simulink model "DvrSimKeybdCircuit_cs_old"  (R2016a)
settings: Solver=ode5  SolverMode=SingleTasking  StartTime=0.0  StopTime=inf  FixedStep=1/1000  RelTol=1e-3
PreLoadFcn:
  | mbxruntime.callbacks.PreLoadFcn(bdroot);
PostLoadFcn:
  | mbxruntime.callbacks.PostLoadFcn(bdroot);
InitFcn:
  | mbxruntime.callbacks.InitFcn(bdroot);
StartFcn:
  | mbxruntime.callbacks.StartFcn(bdroot);
StopFcn:
  | mbxruntime.callbacks.StopFcn(bdroot);
model workspace (MAT data in the model file):
  mbox_table : struct (value not decoded)
  model_closed = 0
  sim_status = 0
undefined symbols (not defined in the file or in its folder): BMotor1, BMotor2, BrkDelayTime, DControlB, Delay1, Delay2, DiscIntNeverNeededParam, IControlB, JMotor1, JMotor2, PControlB, PreScanCarSimLoadFcn, ratioGearF, ratioGearR, TorqDelayTime, Tstep
undefined symbols (not defined in the file): SteeringColumn, SteeringWheel, WheelL0, WheelL1, WheelR0, WheelR1
libraries: simulink x12, simulink_extras x5, MyLib x3, PreScanSimulinkLibrary x3, Solver_SF x2, pil_lib x1, PreScanUsefulBlocks x1
(part 2 of 9)

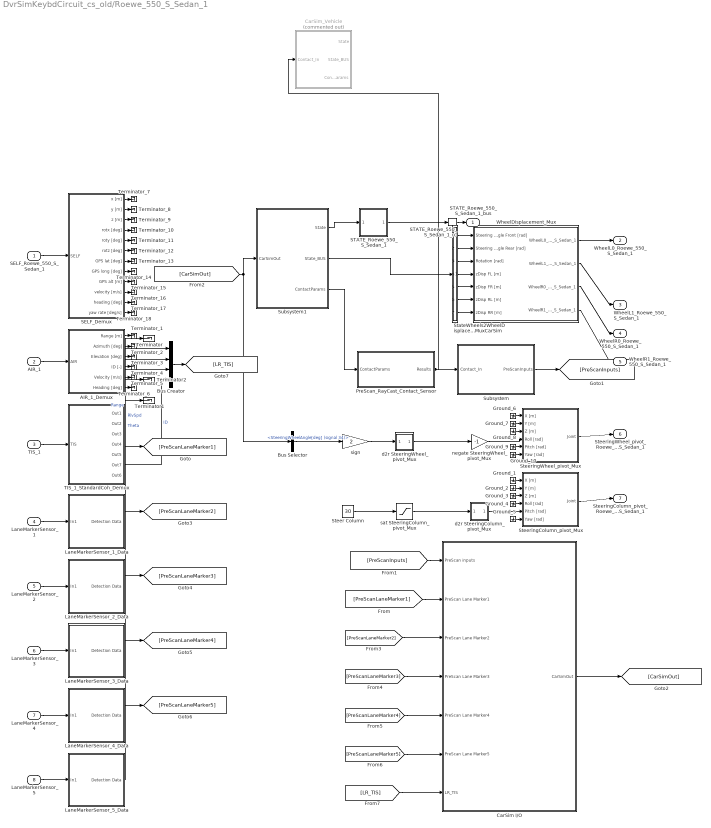
== system DvrSimKeybdCircuit_cs_old/Roewe_550_S_Sedan_1 ==
  SELF_Roewe_550_S_Sedan_1 : Inport  Tag=inport/SelfPort  OutDataTypeStr=Bus: PRESCAN_SELFSENSORDATA  PortDimensions=1  SampleTime=50/1000  BusOutputAsStruct=on
  AIR_1 : Inport  Tag=inport/AIR  Port=2  OutDataTypeStr=Bus: PRESCAN_AIRSENSORMESSAGE  PortDimensions=1  SampleTime=50/1000  BusOutputAsStruct=on
  TIS_1 : Inport  Tag=inport/TIS  Port=3  OutDataTypeStr=Bus: PRESCAN_SCANNERSENSOR_MESSAGE  PortDimensions=1  SampleTime=1/20  BusOutputAsStruct=on
  LaneMarkerSensor_1 : Inport  Tag=inport/LaneMarker  Port=4  OutDataTypeStr=Bus: PRESCAN_LANEMARKER_MESSAGE  PortDimensions=4  SampleTime=1/20  BusOutputAsStruct=on
  LaneMarkerSensor_2 : Inport  Tag=inport/LaneMarker  Port=5  OutDataTypeStr=Bus: PRESCAN_LANEMARKER_MESSAGE  PortDimensions=4  SampleTime=1/20  BusOutputAsStruct=on
  LaneMarkerSensor_3 : Inport  Tag=inport/LaneMarker  Port=6  OutDataTypeStr=Bus: PRESCAN_LANEMARKER_MESSAGE  PortDimensions=4  SampleTime=1/20  BusOutputAsStruct=on
  LaneMarkerSensor_4 : Inport  Tag=inport/LaneMarker  Port=7  OutDataTypeStr=Bus: PRESCAN_LANEMARKER_MESSAGE  PortDimensions=4  SampleTime=1/20  BusOutputAsStruct=on
  LaneMarkerSensor_5 : Inport  Tag=inport/LaneMarker  Port=8  OutDataTypeStr=Bus: PRESCAN_LANEMARKER_MESSAGE  PortDimensions=4  SampleTime=1/20  BusOutputAsStruct=on
  AIR_1_Demux : Subsystem  Tag=demux/AIR  mask(PreScan Demux Block: AIR){DetectionType=Center, detectableObjects=1}
      mask prompts: DetectionType "Detection Type"; detectableObjects "Max. detectable objects"
      mask help:
      | The Actor Information Receiver sensor provides a fast, simple and generic detection solution which is not tied up to a specific technology and can be used for scenarios in which a simple sensor is needed.
      |
      | For more information, please click Help.
      mask init:
      | switch DetectionType
      |     case 1
      |         DetectionTypeStr = 'Center';
      |     case 2
      |         DetectionTypeStr = 'BBox';
      |     case 3
      |         DetectionTypeStr = 'CoG';
      |     otherwise
      |         DetectionTypeStr = 'Unknown';
      | end
      settings: DeleteFcn=PreScanBlockDeleteFcn;
      mask Help: eval('openHelp(413)')
      mask TypeOptions DetectionType: Center | BBox | CoG
      mask Display:
      | disp(char('Det. type:         ',['{\it',DetectionTypeStr,'}']),'texmode','on')
      | port_label('output',1,'Range [m]')
      | port_label('output',2,'{\theta} [deg]','texmode','on')
      | port_label('output',3,'{\phi} [deg]','texmode','on')
      | port_label('output',4,'ID [-]','texmode','on')
      | port_label('output',5,'Velocity [m/s]','texmode','on')
      | port_label('output',6,'Heading [deg]','texmode','on')
  Bus Creator : BusCreator  Inputs=4
  Bus Selector : BusSelector  OutputSignals=SteeringWheelAngle[deg] (signal 34)
  CarSim I/O : Subsystem
  CarSim_Vehicle : Subsystem  Tag=UserSpecified_Subsys  Description=..\..\..\Program Files (x86)\CarSim201601_Data\Extensions\Simulink\CarSim_VehicleDynamics.mdl  Commented=on  LoadFcn=PreScanCarSimLoadFcn();  mask(User specified subsystem){update=off, sourcefilename=..\..\..\Program Files (x86)\CarSim201601_Data\Extensions\Simulink\CarSim_VehicleDynamics.mdl}
      mask prompts: update "Update (default: not checked)"; sourcefilename "Source file name"
      mask help:
      | A User-specified model may be selected as Controller or Dynamics of the vehicle. PreScan will copy the contents of the User-specified model into the user-specified model block.
      |
      | If update checkbox is checked the current user-specified model block will be deleted and will be REPLACED by (new) user specified model blocks. So, the current user specified model elements will be lost.
      |
      | Warning: If a new user-specified model is selected in the GUI, the user-specified model will be replaced.
      settings: DeleteFcn=PreScanBlockDeleteFcn;
      mask Help: eval('openHelp(227)')
      mask Display: userSpecifiedDynamics_mask_display();
  Ground_{1..10} (10 alike) : Ground
  LaneMarkerSensor_1_Data : Subsystem  Tag=demux/LaneMarkerSensor  mask{NUMBEROFSLICES=4, TimeStep=1/20}
      mask prompts: NUMBEROFSLICES "Number of slices"; TimeStep "Auto Assigned: Time Step [s]"
      mask Help: eval('openHelp(2301)')
  LaneMarkerSensor_2_Data : Subsystem  Tag=demux/LaneMarkerSensor  mask{NUMBEROFSLICES=4, TimeStep=1/20}
      mask prompts: NUMBEROFSLICES "Number of slices"; TimeStep "Auto Assigned: Time Step [s]"
      mask Help: eval('openHelp(2301)')
  LaneMarkerSensor_3_Data : Subsystem  Tag=demux/LaneMarkerSensor  mask{NUMBEROFSLICES=4, TimeStep=1/20}
      mask prompts: NUMBEROFSLICES "Number of slices"; TimeStep "Auto Assigned: Time Step [s]"
      mask Help: eval('openHelp(2301)')
  LaneMarkerSensor_4_Data : Subsystem  Tag=demux/LaneMarkerSensor  mask{NUMBEROFSLICES=4, TimeStep=1/20}
      mask prompts: NUMBEROFSLICES "Number of slices"; TimeStep "Auto Assigned: Time Step [s]"
      mask Help: eval('openHelp(2301)')
  LaneMarkerSensor_5_Data : Subsystem  Tag=demux/LaneMarkerSensor  mask{NUMBEROFSLICES=4, TimeStep=1/20}
      mask prompts: NUMBEROFSLICES "Number of slices"; TimeStep "Auto Assigned: Time Step [s]"
      mask Help: eval('openHelp(2301)')
  PreScan_RayCast_Contact_Sensor : Subsystem  Tag=PreScan_RayCast_Contact_Sensor  LoadFcn=|  mask(PreScan Block: PreScan RayCast Contact Sensor){x0=1005.0825, y0=379.7545, z0=1.22, Roll0=0, Pitch0=0, Yaw0=180, wheelRadius=0.44999998807907104, hcog=0.53, b=2.7000000476837158, TimeStep=-1}
      | load PrescanXYZData;
      | load PrescanRPYData;
      | load PrescanQuatData;
      | load PrescanAxisAngleData;
      | load PrescanPoseData;
      | load PrescanPoseQData;
      | load PrescanPoseAData;
      | load PrescanWheelContactData;
      mask prompts: x0 "Ini x-position VEHICLE wrt GLOBAL axis system [m]"; y0 "Ini y-position VEHICLE wrt GLOBAL axis system [m]"; z0 "Ini z-position VEHICLE wrt GLOBAL axis system [m]"; Roll0 "Ini roll-angle BODY wrt VEHICLE axis system [deg]"; Pitch0 "Ini pitch-angle BODY wrt VEHICLE axis system [deg]"; Yaw0 "Ini yaw-angle VEHICLE wrt GLOBAL axis system [deg]"; wheelRadius "Wheel Radius [m]"; hcog "Dynamics: hCoG [m]"; b "Dynamics: b [m]"; TimeStep "Time Step [s]"
      mask help:
      | This block encapsulates the base Contact sensor.
      |
      | It takes input parameters from the PreScan 3D vehicle dynamics block and outputs contact results.
      mask Help: eval('openHelp(251)')
  SELF_Demux : Subsystem  Tag=demux/SelfPort  mask(PreScan Demux Block:){}
      mask help:
      | The SELF port shows (state) information of the actor itself. The outputs are position in the experiment's axis system and the GPS coordinates, and the object's absolute velocity and compass heading.
      |
      | For more information, please click Help.
      settings: DeleteFcn=PreScanBlockDeleteFcn;
      mask Help: eval('openHelp(462)')
      mask Display:
      | port_label('output',1,'x [m]')
      | port_label('output',2,'y [m]')
      | port_label('output',3,'z [m]','texmode','on')
      | port_label('output',4,'Rotx [deg]','texmode','on')
      | port_label('output',5,'Roty [deg]','texmode','on')
      | port_label('output',6,'Rotz [deg]','texmode','on')
      | port_label('output',7,'GPS lat [deg]','texmode','on')
      | port_label('output',8,'GPS long [deg]','texmode','on')
      | port_label('output',9,'GPS alt [m]','texmode','on')
      | port_label('output',10,'Velocity [m/s]')
      | port_label('output',11,'Heading [deg]')
      | port_label('output',12,'Yaw rate [deg/s]')
  STATE_Roewe_550_S_Sedan_1 : Subsystem  Tag=mux/StatePort  Priority=0  LoadFcn=load PrescanStateActuatorData  mask(PreScan Sink Block: State){x0=1005.0825, y0=379.7545, z0=1.22, Roll0=0, Pitch0=0, Yaw0=180, TimeStep=1/1000}
      mask prompts: x0 "Ini x-position VEHICLE wrt GLOBAL axis system [m]"; y0 "Ini y-position VEHICLE wrt GLOBAL axis system [m]"; z0 "Ini z-position VEHICLE wrt GLOBAL axis system [m]"; Roll0 "Ini roll-angle BODY wrt VEHICLE axis system [deg]"; Pitch0 "Ini pitch-angle BODY wrt VEHICLE axis system [deg]"; Yaw0 "Ini yaw-angle VEHICLE wrt GLOBAL axis system [deg]"; TimeStep "Auto-Assigned: Upload Period [s]"
      mask help:
      | The Actor State contains a vector signal of size (9x1), containing the following signals:
      |
      | -  Position                  (x,y,z)                                     [m]
      | -  Velocity                  (vx,vy,vz)                               [m/s]
      | -  Angles                    (Roll, Pitch, Yaw)                   [rad]
      |
      | The Actor state is defined in the global axis system.
      | The state is superponed on the Initial position defined in the GUI.
      |
      | For more information, please click Help.
      settings: DeleteFcn=PreScanBlockDeleteFcn;
      mask Help: eval('openHelp(222)')
      mask Display: image(imread('State.png'))
  STATE_Roewe_550_S_Sedan_1_rc : RateTransition  Tag=mux_rc/StatePort  OutPortSampleTimeOpt=Inherit
  StateWheels2WheelDisplacementMuxCarSim : Subsystem  Tag=StateWheels2WheelDisplacementMuxCarSim  mask(PreScan Utility Block:){}
      mask help: This block selects the CarSim wheels displacement and rotation.
      settings: DeleteFcn=PreScanBlockDeleteFcn;
  Steer Column : Constant  Value=30
  SteeringColumn_pivot_Mux : Subsystem  Tag=mux/Joint  mask(PreScan Mux Block){DisplayName=SteeringColumn}
      mask prompts: DisplayName "Display Name"
      mask help:
      | This block simulates a generic joint used for generic models. This joint can be enabled/disabled from the GUI.
      |
      | For more information, please click Help.
      settings: DeleteFcn=PreScanBlockDeleteFcn;
      mask Help: eval('openHelp(254)')
  SteeringWheel_pivot_Mux : Subsystem  Tag=mux/Joint  mask(PreScan Mux Block){DisplayName=SteeringWheel}
      mask prompts: DisplayName "Display Name"
      mask help:
      | This block simulates a generic joint used for generic models. This joint can be enabled/disabled from the GUI.
      |
      | For more information, please click Help.
      settings: DeleteFcn=PreScanBlockDeleteFcn;
      mask Help: eval('openHelp(254)')
  Subsystem : Subsystem
  Subsystem1 : Subsystem
  TIS_1_StandardCoh_Demux : Subsystem  Tag=demux/TIS/StandardCoh  TreatAsAtomicUnit=on  mask(PreScan Demux Block: TIS){MAXMESSAGES=1}
      mask prompts: MAXMESSAGES "Number of Objects"
      mask Help: eval('openHelp(449)')
      mask Display:
      | port_label('input',1,'TIS')
      | port_label('output',1,'Beam ID [-]')
      | port_label('output',2,'Range [m]')
      | port_label('output',3,'DopplerVelocity [m/s]')
      | port_label('output',4,'{\theta} [deg]','texmode','on')
      | port_label('output',5,'{\phi} [deg]','texmode','on')
      | port_label('output',6,'Target ID [-]','texmode','on')
      | port_label('output',7,'TIS Data','texmode','on')
  Terminator : Terminator
  Terminator1 : Terminator
  Terminator2 : Terminator
  Terminator_{1..18} (18 alike) : Terminator
  WheelDisplacement_Mux : Subsystem  Tag=mux/JointGroup  mask(JointGroup){}
      mask help:
      | The JointGroup allows to control several Joints in one go, as defined for this particular model.
      | For more information, look in the PreScan manual in the section "Model Preparation Tool" -> "Joint Groups"
      |
      | For more information on the Joints simulink interface, press Help.
      mask Help: eval('openHelp(254)')
  d2r SteeringColumn_pivot_Mux : Subsystem  mask(DegreesToRadians){}
      mask help: SimulinkBlocks:simulink_extras:DegreesToRadians_MD
      mask Help: web([docroot '/simulink/ref_extras/degreestoradians.html'])
      mask Display: disp('D2R')
  d2r SteeringWheel_pivot_Mux : Subsystem  mask(DegreesToRadians){}
      mask help: SimulinkBlocks:simulink_extras:DegreesToRadians_MD
      mask Help: web([docroot '/simulink/ref_extras/degreestoradians.html'])
      mask Display: disp('D2R')
  negate SteeringWheel_pivot_Mux : Gain  Gain=-1
  sat SteeringColumn_pivot_Mux : Saturate  UpperLimit=30  LowerLimit=-5
  sign : Gain  Gain=2
  STATE_Roewe_550_S_Sedan_1_bus : Outport  Tag=outport/StatePort  OutDataTypeStr=Bus: PRESCAN_STATEACTUATORDATA  PortDimensions=1  SampleTime=50/1000
  WheelL0_Roewe_550_S_Sedan_1 : Outport  Tag=outport/JointActuator  Port=2  OutDataTypeStr=Bus: PRESCAN_POSE_DATA  SampleTime=50/1000
  WheelL1_Roewe_550_S_Sedan_1 : Outport  Tag=outport/JointActuator  Port=3  OutDataTypeStr=Bus: PRESCAN_POSE_DATA  SampleTime=50/1000
  WheelR0_Roewe_550_S_Sedan_1 : Outport  Tag=outport/JointActuator  Port=4  OutDataTypeStr=Bus: PRESCAN_POSE_DATA  SampleTime=50/1000
  WheelR1_Roewe_550_S_Sedan_1 : Outport  Tag=outport/JointActuator  Port=5  OutDataTypeStr=Bus: PRESCAN_POSE_DATA  SampleTime=50/1000
  SteeringWheel_pivot_Roewe_550_S_Sedan_1 : Outport  Tag=outport/JointActuator  Port=6  OutDataTypeStr=Bus: PRESCAN_POSE_DATA  SampleTime=50/1000
  SteeringColumn_pivot_Roewe_550_S_Sedan_1 : Outport  Tag=outport/JointActuator  Port=7  OutDataTypeStr=Bus: PRESCAN_POSE_DATA  SampleTime=50/1000
  wires:
  LaneMarkerSensor_1_Data/1(Detection Data) -> [PreScanLaneMarker1]
  LaneMarkerSensor_2_Data/1(Detection Data) -> [PreScanLaneMarker2]
  LaneMarkerSensor_3_Data/1(Detection Data) -> [PreScanLaneMarker3]
  LaneMarkerSensor_4_Data/1(Detection Data) -> [PreScanLaneMarker4]
  [PreScanLaneMarker1] -> CarSim I/O/2(PreScan Lane Marker1)
  [PreScanInputs] -> CarSim I/O/1(PreScan inputs)
  Subsystem/1(PreScanInputs) -> [PreScanInputs]
  [CarSimOut] -> Bus Selector/1, Subsystem1/1(CarSimOut)
  PreScan_RayCast_Contact_Sensor/1(Results) -> Subsystem/1(Contact_In), CarSim_Vehicle/1(Contact_In)
  Subsystem1/3(ContactParams) -> PreScan_RayCast_Contact_Sensor/1(ContactParams)
  Subsystem1/1(State) -> STATE_Roewe_550_S_Sedan_1/1(State)
  Subsystem1/2(State_BUS) -> StateWheels2WheelDisplacementMuxCarSim/1(StateWheels)
  CarSim I/O/1(CarSimOut) -> [CarSimOut]
  [PreScanLaneMarker2] -> CarSim I/O/3(PreScan Lane Marker2)
  [PreScanLaneMarker3] -> CarSim I/O/4(PreScan Lane Marker3)
  [PreScanLaneMarker4] -> CarSim I/O/5(PreScan Lane Marker4)
  [PreScanLaneMarker5] -> CarSim I/O/6(PreScan Lane Marker5)
  negate SteeringWheel_pivot_Mux/1 -> SteeringWheel_pivot_Mux/4(Roll [rad])
  d2r SteeringWheel_pivot_Mux/1(Radians out) -> negate SteeringWheel_pivot_Mux/1
  Bus Selector/1 -> sign/1  "<SteeringWheelAngle[deg] (signal 34)>"
  sign/1 -> d2r SteeringWheel_pivot_Mux/1(Degrees in)
  d2r SteeringColumn_pivot_Mux/1(Radians out) -> SteeringColumn_pivot_Mux/5(Pitch [rad])
  sat SteeringColumn_pivot_Mux/1 -> d2r SteeringColumn_pivot_Mux/1(Degrees in)
  Steer Column/1 -> sat SteeringColumn_pivot_Mux/1
  LaneMarkerSensor_5_Data/1(Detection Data) -> [PreScanLaneMarker5]
  TIS_1_StandardCoh_Demux/1(Out1) -> Terminator/1
  TIS_1_StandardCoh_Demux/5(Out5) -> Terminator2/1
  TIS_1_StandardCoh_Demux/7(Out6) -> Terminator1/1
  [LR_TIS] -> CarSim I/O/7(LR_TIS)
  TIS_1_StandardCoh_Demux/2(Out2) -> Bus Creator/1  "Range"
  TIS_1_StandardCoh_Demux/3(Out3) -> Bus Creator/2  "RlvSpd"
  TIS_1_StandardCoh_Demux/4(Out4) -> Bus Creator/3  "Theta"
  TIS_1_StandardCoh_Demux/6(Out7) -> Bus Creator/4  "ID"
  Bus Creator/1 -> [LR_TIS]
  STATE_Roewe_550_S_Sedan_1_rc/1 -> STATE_Roewe_550_S_Sedan_1_bus/1
  STATE_Roewe_550_S_Sedan_1/1(StateBus) -> STATE_Roewe_550_S_Sedan_1_rc/1
  SELF_Roewe_550_S_Sedan_1/1 -> SELF_Demux/1(SELF)
  AIR_1/1 -> AIR_1_Demux/1(AIR)
  TIS_1/1 -> TIS_1_StandardCoh_Demux/1(TIS)
  LaneMarkerSensor_1/1 -> LaneMarkerSensor_1_Data/1(In1)
  LaneMarkerSensor_2/1 -> LaneMarkerSensor_2_Data/1(In1)
  LaneMarkerSensor_3/1 -> LaneMarkerSensor_3_Data/1(In1)
  LaneMarkerSensor_4/1 -> LaneMarkerSensor_4_Data/1(In1)
  LaneMarkerSensor_5/1 -> LaneMarkerSensor_5_Data/1(In1)
  WheelDisplacement_Mux/1(WheelL0_Roewe_550_S_Sedan_1) -> WheelL0_Roewe_550_S_Sedan_1/1
  WheelDisplacement_Mux/2(WheelL1_Roewe_550_S_Sedan_1) -> WheelL1_Roewe_550_S_Sedan_1/1
  WheelDisplacement_Mux/3(WheelR0_Roewe_550_S_Sedan_1) -> WheelR0_Roewe_550_S_Sedan_1/1
  WheelDisplacement_Mux/4(WheelR1_Roewe_550_S_Sedan_1) -> WheelR1_Roewe_550_S_Sedan_1/1
  SteeringWheel_pivot_Mux/1(Joint) -> SteeringWheel_pivot_Roewe_550_S_Sedan_1/1
  SteeringColumn_pivot_Mux/1(Joint) -> SteeringColumn_pivot_Roewe_550_S_Sedan_1/1
  StateWheels2WheelDisplacementMuxCarSim/1(Steering_Angle_Front_[rad]) -> WheelDisplacement_Mux/1(Steering Angle Front [rad])
  StateWheels2WheelDisplacementMuxCarSim/2(Steering_Angle_Rear_[rad]) -> WheelDisplacement_Mux/2(Steering Angle Rear [rad])
  StateWheels2WheelDisplacementMuxCarSim/3(WheelsRotation_[rad]) -> WheelDisplacement_Mux/3(Rotation [rad])
  StateWheels2WheelDisplacementMuxCarSim/4(z displacement FL [m]) -> WheelDisplacement_Mux/4(zDisp FL [m])
  StateWheels2WheelDisplacementMuxCarSim/5(z displacement FR [m]) -> WheelDisplacement_Mux/5(zDisp FR [m])
  StateWheels2WheelDisplacementMuxCarSim/6(z displacement RL [m]) -> WheelDisplacement_Mux/6(zDisp RL [m])
  StateWheels2WheelDisplacementMuxCarSim/7(z displacement RR [m]) -> WheelDisplacement_Mux/7(zDisp RR [m])
  AIR_1_Demux/1(Range [m]) -> Terminator_1/1
  AIR_1_Demux/2(Azimuth [deg]) -> Terminator_2/1
  AIR_1_Demux/3(Elevation [deg]) -> Terminator_3/1
  AIR_1_Demux/4(ID [-]) -> Terminator_4/1
  AIR_1_Demux/5(Velocity [m/s]) -> Terminator_5/1
  AIR_1_Demux/6(Heading [deg]) -> Terminator_6/1
  SELF_Demux/1(x [m]) -> Terminator_7/1
  SELF_Demux/2(y [m]) -> Terminator_8/1
  SELF_Demux/3(z [m]) -> Terminator_9/1
  SELF_Demux/4(rotx [deg]) -> Terminator_10/1
  SELF_Demux/5(roty [deg]) -> Terminator_11/1
  SELF_Demux/6(rotz [deg]) -> Terminator_12/1
  SELF_Demux/7(GPS lat [deg]) -> Terminator_13/1
  SELF_Demux/8(GPS long [deg]) -> Terminator_14/1
  SELF_Demux/9(GPS alt [m]) -> Terminator_15/1
  SELF_Demux/10(velocity [m/s]) -> Terminator_16/1
  SELF_Demux/11(heading [deg]) -> Terminator_17/1
  SELF_Demux/12(yaw rate [deg/s]) -> Terminator_18/1
  Ground_1/1 -> SteeringColumn_pivot_Mux/1(X [m])
  Ground_2/1 -> SteeringColumn_pivot_Mux/2(Y [m])
  Ground_3/1 -> SteeringColumn_pivot_Mux/3(Z [m])
  Ground_4/1 -> SteeringColumn_pivot_Mux/4(Roll [rad])
  Ground_5/1 -> SteeringColumn_pivot_Mux/6(Yaw [rad])
  Ground_6/1 -> SteeringWheel_pivot_Mux/1(X [m])
  Ground_7/1 -> SteeringWheel_pivot_Mux/2(Y [m])
  Ground_8/1 -> SteeringWheel_pivot_Mux/3(Z [m])
  Ground_9/1 -> SteeringWheel_pivot_Mux/5(Pitch [rad])
  Ground_10/1 -> SteeringWheel_pivot_Mux/6(Yaw [rad])

== system DvrSimKeybdCircuit_cs_old/SELF_Roewe_550_S_Sedan_1 ==
  Sensor : S-Function  FunctionName=sfun_SelfSensor  Parameters=UniqueID, TimeStep  SFunctionDeploymentMode=off  EnableBusSupport=off  mask(PreScan Source Block: SELF){UniqueID=29, TimeStep=50/1000}
      mask prompts: UniqueID "Auto-Assigned: Unique ID"; TimeStep "Auto-Assigned: Upload Period [s]"
      mask help:
      | The SELF port shows (state) information of the actor itself. The outputs are position in the experiment's axis system and the GPS coordinates, and the object's absolute velocity and compass heading.
      |
      | For more information, please click Help.
      mask Help: eval('openHelp(462)')
      mask Display: image(imread('GPS.png'))
  SELF_Roewe_550_S_Sedan_1 : Outport  Tag=outport/SelfPort  OutDataTypeStr=Bus: PRESCAN_SELFSENSORDATA  PortDimensions=1  SampleTime=50/1000
  wires:
  Sensor/1 -> SELF_Roewe_550_S_Sedan_1/1

== system DvrSimKeybdCircuit_cs_old/STATE_Roewe_550_S_Sedan_1_bus ==
  STATE_Roewe_550_S_Sedan_1_bus : Inport  Tag=inport/StatePort  OutDataTypeStr=Bus: PRESCAN_STATEACTUATORDATA  PortDimensions=1  SampleTime=50/1000  BusOutputAsStruct=on
  Actuator : S-Function  FunctionName=sfun_StateActuator  Parameters=UniqueID, TimeStep  SFunctionDeploymentMode=off  EnableBusSupport=off  mask(PreScan Sink Block: State){UniqueID=29, TimeStep=50/1000}
      mask prompts: UniqueID "Auto-Assigned: Unique ID"; TimeStep "Auto-Assigned: Upload Period [s]"
      mask help:
      | The Actor State contains a vector signal of size (9x1), containing the following signals:
      |
      | -  Position    	(x,y,z)             	[m]
      | -  Velocity    	(vx,vy,vz)         	[m/s]
      | -  Angles       	(Roll, Pitch, Yaw)	[rad]
      |
      | The Actor state is defined in the global axis system.
      | The state is superponed on the Initial position defined in the GUI.
      |
      | For more information, please click Help.
      mask Help: eval('openHelp(222)')
      mask Display: image(imread('State.png'))
  wires:
  STATE_Roewe_550_S_Sedan_1_bus/1 -> Actuator/1

== system DvrSimKeybdCircuit_cs_old/SteeringColumn_pivot_Roewe_550_S_Sedan_1 ==
  SteeringColumn_pivot_Roewe_550_S_Sedan_1 : Inport  Tag=inport/JointActuator  OutDataTypeStr=Bus: PRESCAN_POSE_DATA  SampleTime=50/1000  BusOutputAsStruct=on
  Actuator : Subsystem  Tag=VisuJoint  mask(PreScan Sink Block: VisuJoint){UniqueID=29, Translate_ObjectID3D=Roewe_550_S_Sedan_1.SteeringColumn_pivot, Rotate_ObjectID3D=Roewe_550_S_Sedan_1.SteeringColumn_pivot, TimeStep=50/1000, DisplayName=[]}
      mask prompts: UniqueID "Parent Unique ID"; Translate_ObjectID3D "Translate Object Name"; Rotate_ObjectID3D "Rotate Object Name"; TimeStep "Simulation Step"; DisplayName "Display Name"
      mask help:
      | The VisuJoint block provides a way to adapt the location and orientation of a part of an object.
      |
      | For more information, please click Help.
      settings: DeleteFcn=PreScanBlockDeleteFcn;
      mask Help: eval('openHelp(223)')
      mask Display: image(imread('Joint.png'))
  wires:
  SteeringColumn_pivot_Roewe_550_S_Sedan_1/1 -> Actuator/1(Joint)

== system DvrSimKeybdCircuit_cs_old/SteeringWheel_pivot_Roewe_550_S_Sedan_1 ==
  SteeringWheel_pivot_Roewe_550_S_Sedan_1 : Inport  Tag=inport/JointActuator  OutDataTypeStr=Bus: PRESCAN_POSE_DATA  SampleTime=50/1000  BusOutputAsStruct=on
  Actuator : Subsystem  Tag=VisuJoint  mask(PreScan Sink Block: VisuJoint){UniqueID=29, Translate_ObjectID3D=Roewe_550_S_Sedan_1.SteeringWheel_pivot, Rotate_ObjectID3D=Roewe_550_S_Sedan_1.SteeringWheel_pivot, TimeStep=50/1000, DisplayName=[]}
      mask prompts: UniqueID "Parent Unique ID"; Translate_ObjectID3D "Translate Object Name"; Rotate_ObjectID3D "Rotate Object Name"; TimeStep "Simulation Step"; DisplayName "Display Name"
      mask help:
      | The VisuJoint block provides a way to adapt the location and orientation of a part of an object.
      |
      | For more information, please click Help.
      settings: DeleteFcn=PreScanBlockDeleteFcn;
      mask Help: eval('openHelp(223)')
      mask Display: image(imread('Joint.png'))
  wires:
  SteeringWheel_pivot_Roewe_550_S_Sedan_1/1 -> Actuator/1(Joint)

== system DvrSimKeybdCircuit_cs_old/Synchronizer ==
  Bus Selector1 : BusSelector  OutputSignals=FederateStopped
  Stop Simulation : Stop
  sfun_Synchronizer : S-Function  FunctionName=sfun_Synchronizer  Parameters=SampleTime  SFunctionDeploymentMode=off  EnableBusSupport=off  mask(Legacy Function){SFunctionSpec=void prescan_synchronizer_outputFcn(void ** work1, PRESCAN_SYNCHRONIZEDATA y1[1]), SampleTime=TimeStep, ShowSpec=on}
      mask prompts: SampleTime "Sample time (-1 for inherited):"; ShowSpec "Display function specification"
      mask help:
      | This block allows you to call the legacy functions specified by the following Legacy Code Tool definition:
      | def.SFunctionName = 'sfun_Synchronizer';
      | def.OutputFcnSpec = 'void prescan_synchronizer_outputFcn(void ** work1, PRESCAN_SYNCHRONIZEDATA y1[1])';
      | def.StartFcnSpec = 'void prescan_synchronizer_startFcn(void ** work1)';
      | def.TerminateFcnSpec = 'void prescan_synchronizer_terminateFcn(void ** work1)';
      | def.HeaderFiles = {'prescan_synchronizer_data.h'};
      | def.HostLibFiles = {'sensorinterfaced.lib'};
      | def.IncPaths = {'src', 'C:\prescandev\vislibrary\vis\..\pimp\include\sensors\InterfaceRTW'};
      | def.SrcPaths = {'src'};
      | def.LibPaths = {'C:\\prescandev\\vislibrary_build\lib'};
      | def.SampleTime = 'parameterized';
      | def.Options.language = 'C';
      mask Help: <p>This block was generated automatically by the Legacy Code Tool. For detailed help on this tool, call<a href="matlab:legacy_code('help')"> legacy_code('help')</a>.</p>
      mask Callback ShowSpec:
      | if strcmp(get_param(gcbh, 'ShowSpec'), 'on')
      |   set_param(gcbh, 'MaskDisplay', sprintf('fprintf(''%s'');', get_param(gcbh, 'SFunctionSpec')));
      | else
      |   set_param(gcbh, 'MaskDisplay', sprintf('fprintf(''%s'');', get_param(gcbh, 'FunctionName')));
      | end
      mask Display: fprintf('void prescan_synchronizer_outputFcn(void ** work1, PRESCAN_SYNCHRONIZEDATA y1[1])');
  wires:
  Bus Selector1/1 -> Stop Simulation/1  "<FederateStopped>"
  sfun_Synchronizer/1 -> Bus Selector1/1

== system DvrSimKeybdCircuit_cs_old/TIS_1 ==
  Sensor : S-Function  FunctionName=sfun_TIS  Parameters=sensorID, detectableObjects, timestep  SFunctionDeploymentMode=off  EnableBusSupport=off  mask(PreScan Source Block: Technology Independent Sensor (TIS)){sensorID=2358, detectableObjects=1, timestep=1/20}
      mask prompts: sensorID "Sensor ID"; detectableObjects "Max detectable objects:"; timestep "MATLAB timestep:"
      mask help:
      | The Technology Independent Sensor (TIS) provides a sensor with all sensor-related influence factors (like noise, drift and accuracy) without being technology specific (like radar and lidar). The TIS detects the closest point on the geometry of an object.
      |
      | For more information, please click Help.
      mask Help: eval('openHelp(449)')
      mask Display: image(imread('TIS.png'))
  TIS_1 : Outport  Tag=outport/TIS  OutDataTypeStr=Bus: PRESCAN_SCANNERSENSOR_MESSAGE  PortDimensions=1  SampleTime=1/20
  wires:
  Sensor/1 -> TIS_1/1

== system DvrSimKeybdCircuit_cs_old/WheelL0_Roewe_550_S_Sedan_1 ==
  WheelL0_Roewe_550_S_Sedan_1 : Inport  Tag=inport/JointActuator  OutDataTypeStr=Bus: PRESCAN_POSE_DATA  SampleTime=50/1000  BusOutputAsStruct=on
  Actuator : Subsystem  Tag=VisuJoint  mask(PreScan Sink Block: VisuJoint){UniqueID=29, Translate_ObjectID3D=Roewe_550_S_Sedan_1.WheelL0, Rotate_ObjectID3D=Roewe_550_S_Sedan_1.WheelL0, TimeStep=50/1000, DisplayName=[]}
      mask prompts: UniqueID "Parent Unique ID"; Translate_ObjectID3D "Translate Object Name"; Rotate_ObjectID3D "Rotate Object Name"; TimeStep "Simulation Step"; DisplayName "Display Name"
      mask help:
      | The VisuJoint block provides a way to adapt the location and orientation of a part of an object.
      |
      | For more information, please click Help.
      settings: DeleteFcn=PreScanBlockDeleteFcn;
      mask Help: eval('openHelp(223)')
      mask Display: image(imread('Joint.png'))
  wires:
  WheelL0_Roewe_550_S_Sedan_1/1 -> Actuator/1(Joint)

== system DvrSimKeybdCircuit_cs_old/WheelL1_Roewe_550_S_Sedan_1 ==
  WheelL1_Roewe_550_S_Sedan_1 : Inport  Tag=inport/JointActuator  OutDataTypeStr=Bus: PRESCAN_POSE_DATA  SampleTime=50/1000  BusOutputAsStruct=on
  Actuator : Subsystem  Tag=VisuJoint  mask(PreScan Sink Block: VisuJoint){UniqueID=29, Translate_ObjectID3D=Roewe_550_S_Sedan_1.WheelL1, Rotate_ObjectID3D=Roewe_550_S_Sedan_1.WheelL1, TimeStep=50/1000, DisplayName=[]}
      mask prompts: UniqueID "Parent Unique ID"; Translate_ObjectID3D "Translate Object Name"; Rotate_ObjectID3D "Rotate Object Name"; TimeStep "Simulation Step"; DisplayName "Display Name"
      mask help:
      | The VisuJoint block provides a way to adapt the location and orientation of a part of an object.
      |
      | For more information, please click Help.
      settings: DeleteFcn=PreScanBlockDeleteFcn;
      mask Help: eval('openHelp(223)')
      mask Display: image(imread('Joint.png'))
  wires:
  WheelL1_Roewe_550_S_Sedan_1/1 -> Actuator/1(Joint)

== system DvrSimKeybdCircuit_cs_old/WheelR0_Roewe_550_S_Sedan_1 ==
  WheelR0_Roewe_550_S_Sedan_1 : Inport  Tag=inport/JointActuator  OutDataTypeStr=Bus: PRESCAN_POSE_DATA  SampleTime=50/1000  BusOutputAsStruct=on
  Actuator : Subsystem  Tag=VisuJoint  mask(PreScan Sink Block: VisuJoint){UniqueID=29, Translate_ObjectID3D=Roewe_550_S_Sedan_1.WheelR0, Rotate_ObjectID3D=Roewe_550_S_Sedan_1.WheelR0, TimeStep=50/1000, DisplayName=[]}
      mask prompts: UniqueID "Parent Unique ID"; Translate_ObjectID3D "Translate Object Name"; Rotate_ObjectID3D "Rotate Object Name"; TimeStep "Simulation Step"; DisplayName "Display Name"
      mask help:
      | The VisuJoint block provides a way to adapt the location and orientation of a part of an object.
      |
      | For more information, please click Help.
      settings: DeleteFcn=PreScanBlockDeleteFcn;
      mask Help: eval('openHelp(223)')
      mask Display: image(imread('Joint.png'))
  wires:
  WheelR0_Roewe_550_S_Sedan_1/1 -> Actuator/1(Joint)

== system DvrSimKeybdCircuit_cs_old/WheelR1_Roewe_550_S_Sedan_1 ==
  WheelR1_Roewe_550_S_Sedan_1 : Inport  Tag=inport/JointActuator  OutDataTypeStr=Bus: PRESCAN_POSE_DATA  SampleTime=50/1000  BusOutputAsStruct=on
  Actuator : Subsystem  Tag=VisuJoint  mask(PreScan Sink Block: VisuJoint){UniqueID=29, Translate_ObjectID3D=Roewe_550_S_Sedan_1.WheelR1, Rotate_ObjectID3D=Roewe_550_S_Sedan_1.WheelR1, TimeStep=50/1000, DisplayName=[]}
      mask prompts: UniqueID "Parent Unique ID"; Translate_ObjectID3D "Translate Object Name"; Rotate_ObjectID3D "Rotate Object Name"; TimeStep "Simulation Step"; DisplayName "Display Name"
      mask help:
      | The VisuJoint block provides a way to adapt the location and orientation of a part of an object.
      |
      | For more information, please click Help.
      settings: DeleteFcn=PreScanBlockDeleteFcn;
      mask Help: eval('openHelp(223)')
      mask Display: image(imread('Joint.png'))
  wires:
  WheelR1_Roewe_550_S_Sedan_1/1 -> Actuator/1(Joint)

== system DvrSimKeybdCircuit_cs_old/Roewe_550_S_Sedan_1/AIR_1_Demux ==
  AIR : Inport
  Activate_Switch : Subsystem
      mask Display: text(5,10,'')
  Bus Selector : BusSelector  OutputSignals=DATA.Range,DATA.Azimuth,DATA.Elevation,DATA.ID,DATA.Velocity,DATA.Heading
  Data Type Conversion : DataTypeConversion  OutDataTypeStr=double
  For Iterator : ForIterator  ResetStates=reset  IterationLimit=detectableObjects
  Selector : Selector  InputPortWidth=detectableObjects  IndexOptions=Index vector (port)  Indices=[1 3]  OutputSizes=1
  Signal2ArrayOfSignals1 : Subsystem  mask{VECTORLENGTH=detectableObjects}
      mask prompts: VECTORLENGTH "Length of vector"
  Signal2ArrayOfSignals2 : Subsystem  mask{VECTORLENGTH=detectableObjects}
      mask prompts: VECTORLENGTH "Length of vector"
  Signal2ArrayOfSignals3 : Subsystem  mask{VECTORLENGTH=detectableObjects}
      mask prompts: VECTORLENGTH "Length of vector"
  Signal2ArrayOfSignals4 : Subsystem  mask{VECTORLENGTH=detectableObjects}
      mask prompts: VECTORLENGTH "Length of vector"
  Signal2ArrayOfSignals5 : Subsystem  mask{VECTORLENGTH=detectableObjects}
      mask prompts: VECTORLENGTH "Length of vector"
  Signal2ArrayOfSignals6 : Subsystem  mask{VECTORLENGTH=detectableObjects}
      mask prompts: VECTORLENGTH "Length of vector"
  Range [m] : Outport
  Azimuth [deg] : Outport  Port=2
  Elevation [deg] : Outport  Port=3
  ID [-] : Outport  Port=4
  Velocity [m/s] : Outport  Port=5
  Heading [deg] : Outport  Port=6
  wires:
  Data Type Conversion/1 -> ID [-]/1
  Bus Selector/6 -> Signal2ArrayOfSignals6/2(Element)  "<Heading>"
  Signal2ArrayOfSignals6/1(ArrayofElements) -> Activate_Switch/2(Heading)
  Bus Selector/5 -> Signal2ArrayOfSignals5/2(Element)  "<Velocity>"
  Signal2ArrayOfSignals5/1(ArrayofElements) -> Velocity [m/s]/1
  Bus Selector/4 -> Signal2ArrayOfSignals4/2(Element)  "<ID>"
  Signal2ArrayOfSignals4/1(ArrayofElements) -> Data Type Conversion/1, Activate_Switch/1(BeamID)
  Bus Selector/3 -> Signal2ArrayOfSignals3/2(Element)  "<Elevation>"
  Signal2ArrayOfSignals3/1(ArrayofElements) -> Elevation [deg]/1
  Bus Selector/2 -> Signal2ArrayOfSignals1/2(Element)  "<Azimuth>"
  Signal2ArrayOfSignals1/1(ArrayofElements) -> Azimuth [deg]/1
  Signal2ArrayOfSignals2/1(ArrayofElements) -> Range [m]/1
  Bus Selector/1 -> Signal2ArrayOfSignals2/2(Element)  "<Range>"
  Selector/1 -> Bus Selector/1
  For Iterator/1 -> Signal2ArrayOfSignals6/1(LoopIndex), Signal2ArrayOfSignals5/1(LoopIndex), Signal2ArrayOfSignals4/1(LoopIndex), Signal2ArrayOfSignals3/1(LoopIndex), Signal2ArrayOfSignals1/1(LoopIndex), Signal2ArrayOfSignals2/1(LoopIndex), Selector/2
  AIR/1 -> Selector/1
  Activate_Switch/1(On/Off) -> Heading [deg]/1

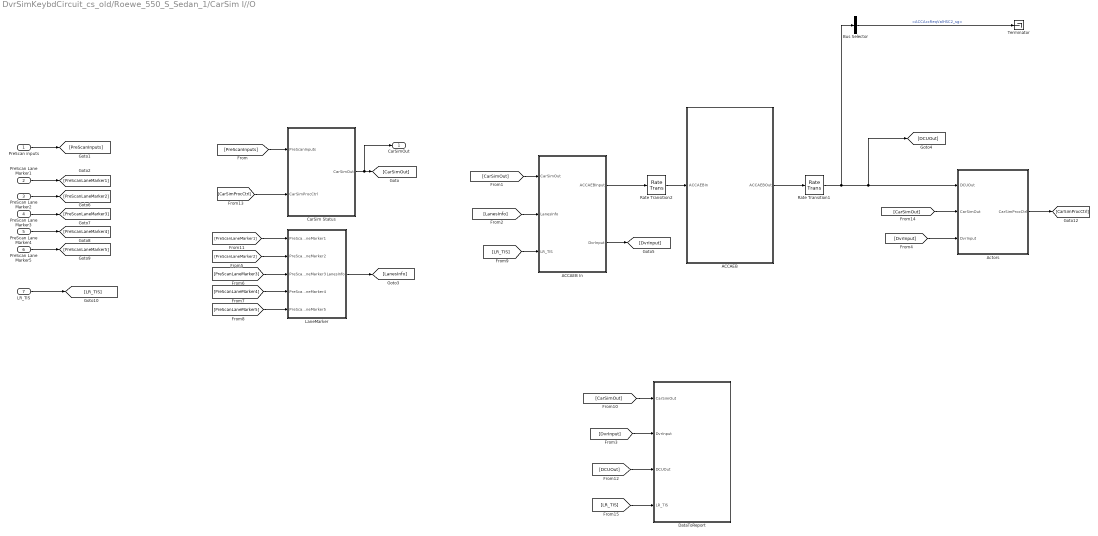
== system DvrSimKeybdCircuit_cs_old/Roewe_550_S_Sedan_1/CarSim I//O ==
  PreScan inputs : Inport
  PreScan Lane Marker1 : Inport  Port=2
  PreScan Lane Marker2 : Inport  Port=3
  PreScan Lane Marker3 : Inport  Port=4
  PreScan Lane Marker4 : Inport  Port=5
  PreScan Lane Marker5 : Inport  Port=6
  LR_TIS : Inport  Port=7
  ACCAEB : Subsystem  DialogController=pil_create_dialog  LoadFcn=|
      | try
      |    if ~strcmp(rtw.pil.getPILVersion, '6.10 (R2016a)_12')
      |       set_param(gcb, 'DialogController', '');
      |       set_param(gcb, 'DialogControllerArgs', '');
      |    end
      | catch e
      |       set_param(gcb, 'DialogController', '');
      |       set_param(gcb, 'DialogControllerArgs', '');
      | end
      mask help: PIL:pil:XILBlockMaskDesc
      mask Display: disp('SIL S-Function');
  ACCAEB In : Subsystem  TreatAsAtomicUnit=on
  Actors : Subsystem
  Bus Selector : BusSelector  OutputSignals=ACCAccReqValHSC2_sg
  "CarSim Status " : Subsystem  TreatAsAtomicUnit=on
  DataToReport : Subsystem  TreatAsAtomicUnit=on  SystemSampleTime=0.05
  LaneMarker : Subsystem  TreatAsAtomicUnit=on  SystemSampleTime=0.1
  Rate Transition1 : RateTransition  OutPortSampleTime=0.001
  Rate Transition2 : RateTransition  OutPortSampleTime=0.01
  Terminator : Terminator
  CarSimOut : Outport
  wires:
  [PreScanInputs] -> "CarSim Status "/1(PreScanInputs)
  PreScan inputs/1 -> [PreScanInputs]
  PreScan Lane Marker1/1 -> [PreScanLaneMarker1]
  "CarSim Status "/1(CarSimOut) -> CarSimOut/1, [CarSimOut]
  [CarSimOut] -> ACCAEB In/1(CarSimOut)
  [LanesInfo] -> ACCAEB In/2(LanesInfo)
  [LR_TIS] -> ACCAEB In/3(LR_TIS)
  [CarSimProcCtrl] -> "CarSim Status "/2(CarSimProcCtrl)
  PreScan Lane Marker2/1 -> [PreScanLaneMarker2]
  PreScan Lane Marker3/1 -> [PreScanLaneMarker3]
  PreScan Lane Marker4/1 -> [PreScanLaneMarker4]
  PreScan Lane Marker5/1 -> [PreScanLaneMarker5]
  Rate Transition2/1 -> ACCAEB/1(ACCAEBIn)
  ACCAEB In/1(ACCAEBInput) -> Rate Transition2/1
  ACCAEB/1(ACCAEBOut) -> Rate Transition1/1
  Rate Transition1/1 -> Bus Selector/1, [DCUOut], Actors/1(DCUOut)
  [CarSimOut] -> Actors/2(CarSimOut)
  Actors/1(CarSimProcCtrl) -> [CarSimProcCtrl]
  ACCAEB In/2(DvrInput) -> [DvrInput]
  [DvrInput] -> Actors/3(DvrInput)
  LaneMarker/1(LanesInfo) -> [LanesInfo]
  [PreScanLaneMarker4] -> LaneMarker/4(PreScanLaneMarker4)
  [PreScanLaneMarker3] -> LaneMarker/3(PreScanLaneMarker3)
  [PreScanLaneMarker5] -> LaneMarker/5(PreScanLaneMarker5)
  [PreScanLaneMarker2] -> LaneMarker/2(PreScanLaneMarker2)
  [PreScanLaneMarker1] -> LaneMarker/1(PreScanLaneMarker1)
  LR_TIS/1 -> [LR_TIS]
  Bus Selector/1 -> Terminator/1  "<ACCAccReqValHSC2_sg>"
  [DvrInput] -> DataToReport/2(DvrInput)
  [CarSimOut] -> DataToReport/1(CarSimOut)
  [DCUOut] -> DataToReport/3(DCUOut)
  [LR_TIS] -> DataToReport/4(LR_TIS)

== system DvrSimKeybdCircuit_cs_old/Roewe_550_S_Sedan_1/CarSim_Vehicle ==
  note: For state mode 'Dynamic' positions
      | are not taken into account, as they
      | are computed by integrating velocity.
      | Click annotation for Help.
  Contact_In : Inport
  CarSim S-Function2 : Solver_SF/CarSim S-Function2  Priority=1  VehicleCode=i_i  SIMFILE=simfile.sim
      settings: AttributesFormatString=Vehicle Code: %<VehicleCode>
  CarSim2PreScanSTATE : Subsystem  Tag=CarSim2PreScanSTATE  mask(CarSim2PreScan:){z0=1.22}
      mask prompts: z0 "PreScan Actor initial COG z-position wrt GLOBAL axis system [m]"
      mask help: This block converts the outputs coming from the CarSim block into consistent PreScan signals.
  CarSim2PreScan_BUS : Subsystem  Tag=CarSim2PreScan_BUS  mask(PreScan block: CarSim to PreScan BUS){TyreRadius=0.44999998807907104, cogZOffset=0.53}
      mask prompts: TyreRadius "Tyre Radius [m]"; cogZOffset "cog Z offset [m]"
      mask help: CarSim to PreScan BUS selector
      mask Help: eval('openHelp()')
      mask Display: disp('PreScan BUS\nVehicleDynamics')
  CarSim2PreScan_ContactAdapter : Subsystem  Tag=CarSim2PreScan_ContactAdapter  mask{wheelRadius=0.44999998807907104}
      mask prompts: wheelRadius "Wheel radius:"
  MuxState : Subsystem  Tag=mux/State  mask(Empty Dynamics State Block){positioningmode=on, TimeStep=1/1000}
      mask prompts: positioningmode "Positioning Mode"; TimeStep "Auto Assigned: Time Step [s]"
      mask help:
      | Build the state of an actor based on user input.
      | The user can either use positioning mode or dynamics mode.
      | - When using positioning mode the position and orientation of the actor are set directly based on the input. Expected input is relative to the initial position and orientation of the actor. It's also possible to specify the velocity of the actor, though this input isn't used, only passed on.
      | - When using dynamics mode the position input is ignored. Expected input is velocity and orientation. The velocity is relative the current orientation of the actor, while orientation is relative to its initial orientation. The position of the actor is calculated based on the velocity and orientation given.
      settings: DeleteFcn=PreScanBlockDeleteFcn;
  TyreContact To Road Information : Subsystem  Tag=TyreContactToRoadInformation  mask{Roll0=0, Pitch0=0, Yaw0=180}
      mask prompts: Roll0 "Ini roll-angle BODY wrt VEHICLE axis system [deg]"; Pitch0 "Ini pitch-angle BODY wrt VEHICLE axis system [deg]"; Yaw0 "Ini yaw-angle VEHICLE wrt GLOBAL axis system [deg]"
  State : Outport
  State_BUS : Outport  Port=2
  ContactParams : Outport  Port=3
  wires:
  MuxState/1(state) -> State/1, CarSim2PreScan_ContactAdapter/1(State)
  CarSim2PreScanSTATE/1(x [m]) -> MuxState/1(x [m])
  CarSim2PreScanSTATE/2(y [m]) -> MuxState/2(y [m])
  CarSim2PreScanSTATE/3(z [m]) -> MuxState/3(z [m])
  CarSim2PreScanSTATE/4(dx [m/s]) -> MuxState/4(dx [m/s])
  CarSim2PreScanSTATE/5(dy [m/s]) -> MuxState/5(dy [m/s])
  CarSim2PreScanSTATE/6(dz [m/s]) -> MuxState/6(dz [m/s])
  CarSim2PreScanSTATE/7(R [rad]) -> MuxState/7(R [rad])
  CarSim2PreScanSTATE/8(P [rad]) -> MuxState/8(P [rad])
  CarSim2PreScanSTATE/9(Y [rad]) -> MuxState/9(Y [rad])
  CarSim2PreScan_BUS/1(PreScanBUS_VehicleDynamics) -> State_BUS/1, CarSim2PreScan_ContactAdapter/2(State_Bus)
  CarSim S-Function2/1 -> CarSim2PreScanSTATE/1(CarSim_In), CarSim2PreScan_BUS/1(CarSim_In)
  Contact_In/1 -> TyreContact To Road Information/1(TyreInfo_in)
  CarSim2PreScan_ContactAdapter/1(ContactParams) -> ContactParams/1

== system DvrSimKeybdCircuit_cs_old/Roewe_550_S_Sedan_1/LaneMarkerSensor_1_Data ==
  In1 : Inport
  Bus Creator : BusCreator  Inputs='SliceCount','ScanAtSensor','ScanAtDistance1','ScanAtDistance2','ScanAtDistance3'
  Constant : Constant
  Constant1 : Constant  Value=NUMBEROFSLICES
  Constant2 : Constant  Value=2
  Constant3 : Constant  Value=3
  Constant4 : Constant  Value=4
  Data Type Conversion : DataTypeConversion  OutDataTypeStr=int32
  If{,1..3} (4 alike) : If  NumInputs=2  IfExpression=u1 >= u2  ShowElse=off
  If Action Subsystem1 : Subsystem  TreatAsAtomicUnit=on
  If Action Subsystem2 : Subsystem  TreatAsAtomicUnit=on
  If Action Subsystem3 : Subsystem  TreatAsAtomicUnit=on
  If Action Subsystem4 : Subsystem  TreatAsAtomicUnit=on
  Merge{,1..3} (4 alike) : Merge  InitialOutput=0
  Zero-filled data bus{,1..3} (4 alike) : Constant  Value=0  VectorParams1D=off  OutDataTypeStr=Bus: PRESCAN_LANEMARKER_DATA  SampleTime=TimeStep
  Detection Data : Outport
  wires:
  Data Type Conversion/1 -> Bus Creator/1  "SliceCount"
  In1/1 -> If Action Subsystem2/1(In1), If Action Subsystem4/1(In1), If Action Subsystem3/1(In1), If Action Subsystem1/1(In1)
  Zero-filled data bus3/1 -> Merge3/1
  Zero-filled data bus2/1 -> Merge2/1
  Zero-filled data bus1/1 -> Merge1/1
  Zero-filled data bus/1 -> Merge/1
  Merge3/1 -> Bus Creator/5  "ScanAtDistance3"
  Merge2/1 -> Bus Creator/4  "ScanAtDistance2"
  Merge1/1 -> Bus Creator/3  "ScanAtDistance1"
  If3/1 -> If Action Subsystem4/Action
  If Action Subsystem4/1(Out1) -> Merge3/2
  Constant4/1 -> If3/2, If Action Subsystem4/2(In2)
  If2/1 -> If Action Subsystem3/Action
  If Action Subsystem3/1(Out1) -> Merge2/2
  Constant3/1 -> If Action Subsystem3/2(In2), If2/2
  If1/1 -> If Action Subsystem1/Action
  If Action Subsystem1/1(Out1) -> Merge1/2
  Constant2/1 -> If Action Subsystem1/2(In2), If1/2
  Merge/1 -> Bus Creator/2  "ScanAtSensor"
  Bus Creator/1 -> Detection Data/1
  If/1 -> If Action Subsystem2/Action
  If Action Subsystem2/1(Out1) -> Merge/2
  Constant/1 -> If Action Subsystem2/2(In2), If/2
  Constant1/1 -> Data Type Conversion/1, If3/1, If2/1, If1/1, If/1

== system DvrSimKeybdCircuit_cs_old/Roewe_550_S_Sedan_1/LaneMarkerSensor_2_Data ==
  In1 : Inport
  Bus Creator : BusCreator  Inputs='SliceCount','ScanAtSensor','ScanAtDistance1','ScanAtDistance2','ScanAtDistance3'
  Constant : Constant
  Constant1 : Constant  Value=NUMBEROFSLICES
  Constant2 : Constant  Value=2
  Constant3 : Constant  Value=3
  Constant4 : Constant  Value=4
  Data Type Conversion : DataTypeConversion  OutDataTypeStr=int32
  If{,1..3} (4 alike) : If  NumInputs=2  IfExpression=u1 >= u2  ShowElse=off
  If Action Subsystem1 : Subsystem  TreatAsAtomicUnit=on
  If Action Subsystem2 : Subsystem  TreatAsAtomicUnit=on
  If Action Subsystem3 : Subsystem  TreatAsAtomicUnit=on
  If Action Subsystem4 : Subsystem  TreatAsAtomicUnit=on
  Merge{,1..3} (4 alike) : Merge  InitialOutput=0
  Zero-filled data bus{,1..3} (4 alike) : Constant  Value=0  VectorParams1D=off  OutDataTypeStr=Bus: PRESCAN_LANEMARKER_DATA  SampleTime=TimeStep
  Detection Data : Outport
  wires:
  Data Type Conversion/1 -> Bus Creator/1  "SliceCount"
  In1/1 -> If Action Subsystem2/1(In1), If Action Subsystem4/1(In1), If Action Subsystem3/1(In1), If Action Subsystem1/1(In1)
  Zero-filled data bus3/1 -> Merge3/1
  Zero-filled data bus2/1 -> Merge2/1
  Zero-filled data bus1/1 -> Merge1/1
  Zero-filled data bus/1 -> Merge/1
  Merge3/1 -> Bus Creator/5  "ScanAtDistance3"
  Merge2/1 -> Bus Creator/4  "ScanAtDistance2"
  Merge1/1 -> Bus Creator/3  "ScanAtDistance1"
  If3/1 -> If Action Subsystem4/Action
  If Action Subsystem4/1(Out1) -> Merge3/2
  Constant4/1 -> If3/2, If Action Subsystem4/2(In2)
  If2/1 -> If Action Subsystem3/Action
  If Action Subsystem3/1(Out1) -> Merge2/2
  Constant3/1 -> If Action Subsystem3/2(In2), If2/2
  If1/1 -> If Action Subsystem1/Action
  If Action Subsystem1/1(Out1) -> Merge1/2
  Constant2/1 -> If Action Subsystem1/2(In2), If1/2
  Merge/1 -> Bus Creator/2  "ScanAtSensor"
  Bus Creator/1 -> Detection Data/1
  If/1 -> If Action Subsystem2/Action
  If Action Subsystem2/1(Out1) -> Merge/2
  Constant/1 -> If Action Subsystem2/2(In2), If/2
  Constant1/1 -> Data Type Conversion/1, If3/1, If2/1, If1/1, If/1

== system DvrSimKeybdCircuit_cs_old/Roewe_550_S_Sedan_1/LaneMarkerSensor_3_Data ==
  In1 : Inport
  Bus Creator : BusCreator  Inputs='SliceCount','ScanAtSensor','ScanAtDistance1','ScanAtDistance2','ScanAtDistance3'
  Constant : Constant
  Constant1 : Constant  Value=NUMBEROFSLICES
  Constant2 : Constant  Value=2
  Constant3 : Constant  Value=3
  Constant4 : Constant  Value=4
  Data Type Conversion : DataTypeConversion  OutDataTypeStr=int32
  If{,1..3} (4 alike) : If  NumInputs=2  IfExpression=u1 >= u2  ShowElse=off
  If Action Subsystem1 : Subsystem  TreatAsAtomicUnit=on
  If Action Subsystem2 : Subsystem  TreatAsAtomicUnit=on
  If Action Subsystem3 : Subsystem  TreatAsAtomicUnit=on
  If Action Subsystem4 : Subsystem  TreatAsAtomicUnit=on
  Merge{,1..3} (4 alike) : Merge  InitialOutput=0
  Zero-filled data bus{,1..3} (4 alike) : Constant  Value=0  VectorParams1D=off  OutDataTypeStr=Bus: PRESCAN_LANEMARKER_DATA  SampleTime=TimeStep
  Detection Data : Outport
  wires:
  Data Type Conversion/1 -> Bus Creator/1  "SliceCount"
  In1/1 -> If Action Subsystem2/1(In1), If Action Subsystem4/1(In1), If Action Subsystem3/1(In1), If Action Subsystem1/1(In1)
  Zero-filled data bus3/1 -> Merge3/1
  Zero-filled data bus2/1 -> Merge2/1
  Zero-filled data bus1/1 -> Merge1/1
  Zero-filled data bus/1 -> Merge/1
  Merge3/1 -> Bus Creator/5  "ScanAtDistance3"
  Merge2/1 -> Bus Creator/4  "ScanAtDistance2"
  Merge1/1 -> Bus Creator/3  "ScanAtDistance1"
  If3/1 -> If Action Subsystem4/Action
  If Action Subsystem4/1(Out1) -> Merge3/2
  Constant4/1 -> If3/2, If Action Subsystem4/2(In2)
  If2/1 -> If Action Subsystem3/Action
  If Action Subsystem3/1(Out1) -> Merge2/2
  Constant3/1 -> If Action Subsystem3/2(In2), If2/2
  If1/1 -> If Action Subsystem1/Action
  If Action Subsystem1/1(Out1) -> Merge1/2
  Constant2/1 -> If Action Subsystem1/2(In2), If1/2
  Merge/1 -> Bus Creator/2  "ScanAtSensor"
  Bus Creator/1 -> Detection Data/1
  If/1 -> If Action Subsystem2/Action
  If Action Subsystem2/1(Out1) -> Merge/2
  Constant/1 -> If Action Subsystem2/2(In2), If/2
  Constant1/1 -> Data Type Conversion/1, If3/1, If2/1, If1/1, If/1

== system DvrSimKeybdCircuit_cs_old/Roewe_550_S_Sedan_1/LaneMarkerSensor_4_Data ==
  In1 : Inport
  Bus Creator : BusCreator  Inputs='SliceCount','ScanAtSensor','ScanAtDistance1','ScanAtDistance2','ScanAtDistance3'
  Constant : Constant
  Constant1 : Constant  Value=NUMBEROFSLICES
  Constant2 : Constant  Value=2
  Constant3 : Constant  Value=3
  Constant4 : Constant  Value=4
  Data Type Conversion : DataTypeConversion  OutDataTypeStr=int32
  If{,1..3} (4 alike) : If  NumInputs=2  IfExpression=u1 >= u2  ShowElse=off
  If Action Subsystem1 : Subsystem  TreatAsAtomicUnit=on
  If Action Subsystem2 : Subsystem  TreatAsAtomicUnit=on
  If Action Subsystem3 : Subsystem  TreatAsAtomicUnit=on
  If Action Subsystem4 : Subsystem  TreatAsAtomicUnit=on
  Merge{,1..3} (4 alike) : Merge  InitialOutput=0
  Zero-filled data bus{,1..3} (4 alike) : Constant  Value=0  VectorParams1D=off  OutDataTypeStr=Bus: PRESCAN_LANEMARKER_DATA  SampleTime=TimeStep
  Detection Data : Outport
  wires:
  Data Type Conversion/1 -> Bus Creator/1  "SliceCount"
  In1/1 -> If Action Subsystem2/1(In1), If Action Subsystem4/1(In1), If Action Subsystem3/1(In1), If Action Subsystem1/1(In1)
  Zero-filled data bus3/1 -> Merge3/1
  Zero-filled data bus2/1 -> Merge2/1
  Zero-filled data bus1/1 -> Merge1/1
  Zero-filled data bus/1 -> Merge/1
  Merge3/1 -> Bus Creator/5  "ScanAtDistance3"
  Merge2/1 -> Bus Creator/4  "ScanAtDistance2"
  Merge1/1 -> Bus Creator/3  "ScanAtDistance1"
  If3/1 -> If Action Subsystem4/Action
  If Action Subsystem4/1(Out1) -> Merge3/2
  Constant4/1 -> If3/2, If Action Subsystem4/2(In2)
  If2/1 -> If Action Subsystem3/Action
  If Action Subsystem3/1(Out1) -> Merge2/2
  Constant3/1 -> If Action Subsystem3/2(In2), If2/2
  If1/1 -> If Action Subsystem1/Action
  If Action Subsystem1/1(Out1) -> Merge1/2
  Constant2/1 -> If Action Subsystem1/2(In2), If1/2
  Merge/1 -> Bus Creator/2  "ScanAtSensor"
  Bus Creator/1 -> Detection Data/1
  If/1 -> If Action Subsystem2/Action
  If Action Subsystem2/1(Out1) -> Merge/2
  Constant/1 -> If Action Subsystem2/2(In2), If/2
  Constant1/1 -> Data Type Conversion/1, If3/1, If2/1, If1/1, If/1

== system DvrSimKeybdCircuit_cs_old/Roewe_550_S_Sedan_1/LaneMarkerSensor_5_Data ==
  In1 : Inport
  Bus Creator : BusCreator  Inputs='SliceCount','ScanAtSensor','ScanAtDistance1','ScanAtDistance2','ScanAtDistance3'
  Constant : Constant
  Constant1 : Constant  Value=NUMBEROFSLICES
  Constant2 : Constant  Value=2
  Constant3 : Constant  Value=3
  Constant4 : Constant  Value=4
  Data Type Conversion : DataTypeConversion  OutDataTypeStr=int32
  If{,1..3} (4 alike) : If  NumInputs=2  IfExpression=u1 >= u2  ShowElse=off
  If Action Subsystem1 : Subsystem  TreatAsAtomicUnit=on
  If Action Subsystem2 : Subsystem  TreatAsAtomicUnit=on
  If Action Subsystem3 : Subsystem  TreatAsAtomicUnit=on
  If Action Subsystem4 : Subsystem  TreatAsAtomicUnit=on
  Merge{,1..3} (4 alike) : Merge  InitialOutput=0
  Zero-filled data bus{,1..3} (4 alike) : Constant  Value=0  VectorParams1D=off  OutDataTypeStr=Bus: PRESCAN_LANEMARKER_DATA  SampleTime=TimeStep
  Detection Data : Outport
  wires:
  Data Type Conversion/1 -> Bus Creator/1  "SliceCount"
  In1/1 -> If Action Subsystem2/1(In1), If Action Subsystem4/1(In1), If Action Subsystem3/1(In1), If Action Subsystem1/1(In1)
  Zero-filled data bus3/1 -> Merge3/1
  Zero-filled data bus2/1 -> Merge2/1
  Zero-filled data bus1/1 -> Merge1/1
  Zero-filled data bus/1 -> Merge/1
  Merge3/1 -> Bus Creator/5  "ScanAtDistance3"
  Merge2/1 -> Bus Creator/4  "ScanAtDistance2"
  Merge1/1 -> Bus Creator/3  "ScanAtDistance1"
  If3/1 -> If Action Subsystem4/Action
  If Action Subsystem4/1(Out1) -> Merge3/2
  Constant4/1 -> If3/2, If Action Subsystem4/2(In2)
  If2/1 -> If Action Subsystem3/Action
  If Action Subsystem3/1(Out1) -> Merge2/2
  Constant3/1 -> If Action Subsystem3/2(In2), If2/2
  If1/1 -> If Action Subsystem1/Action
  If Action Subsystem1/1(Out1) -> Merge1/2
  Constant2/1 -> If Action Subsystem1/2(In2), If1/2
  Merge/1 -> Bus Creator/2  "ScanAtSensor"
  Bus Creator/1 -> Detection Data/1
  If/1 -> If Action Subsystem2/Action
  If Action Subsystem2/1(Out1) -> Merge/2
  Constant/1 -> If Action Subsystem2/2(In2), If/2
  Constant1/1 -> Data Type Conversion/1, If3/1, If2/1, If1/1, If/1
